simulink library "TQR_lib"  (Simulink 7.5)
settings: Solver=ode45  StartTime=0.0  StopTime=10.0  RelTol=1e-3
values from neighbouring files (symbols this model uses):
  p1_ACPI_PICFilDen1_na = Simulink.Parameter    [TQR_par.m]
  p1_ACPI_PICFilDen2_na = Simulink.Parameter    [TQR_par.m]
  p1_ACPI_PICFilDen3_na = Simulink.Parameter    [TQR_par.m]
  p1_ACPI_PICFilNum1_na = Simulink.Parameter    [TQR_par.m]
  p1_ACPI_PICFilNum2_na = Simulink.Parameter    [TQR_par.m]
  p1_ACPI_PICFilNum3_na = Simulink.Parameter    [TQR_par.m]
  pTQR_bar_BrkPOvrdRecoverThd_C = Simulink.Parameter    [TQR_par.m]
  pTQR_bar_BrkPOvrdVal_C = Simulink.Parameter    [TQR_par.m]
  pTQR_bar_ECrpTrqStrtPres_C = Simulink.Parameter    [TQR_par.m]
  pTQR_bar_MasterCylPres_CUR = Simulink.Parameter    [TQR_par.m]
  pTQR_bool_AccPedOvrdDsbl_C = Simulink.Parameter    [TQR_par.m]
  pTQR_bool_BrkPOvrdDsbl_C = Simulink.Parameter    [TQR_par.m]
  pTQR_bool_BrkRecupSrcSelSwt_C = Simulink.Parameter    [TQR_par.m]
  pTQR_bool_PICTqEna_C = Simulink.Parameter    [TQR_par.m]
  pTQR_bool_RecupEna_C = Simulink.Parameter    [TQR_par.m]
  pTQR_kmph_MaxVehSpd_C = Simulink.Parameter    [TQR_par.m]
  pTQR_kmph_MinVehSpd_C = Simulink.Parameter    [TQR_par.m]
  pTQR_kmph_VehSpd_TAB = Simulink.Parameter    [TQR_par.m]
  pTQR_kmph_VehSpdMaxDriving_TAB = Simulink.Parameter    [TQR_par.m]
  pTQR_kmph_VehSpdMaxReverse_TAB = Simulink.Parameter    [TQR_par.m]
  pTQR_kmph_VehSpdRednHi_CUR = Simulink.Parameter    [TQR_par.m]
  pTQR_kmph_VehSpdRednLo_CUR = Simulink.Parameter    [TQR_par.m]
  pTQR_Nm_ACCDelyOutTrq_C = Simulink.Parameter    [TQR_par.m]
  pTQR_Nm_ACCOutTrqLo_C = Simulink.Parameter    [TQR_par.m]
  pTQR_Nm_ACCOutTrqUp_C = Simulink.Parameter    [TQR_par.m]
  pTQR_Nm_BrkECrpTrq_TAB = Simulink.Parameter    [TQR_par.m]
  pTQR_Nm_MaxRecupTq_C = Simulink.Parameter    [TQR_par.m]
  pTQR_Nm_MotCtlrMaxTqLim_C = Simulink.Parameter    [TQR_par.m]
  pTQR_Nm_MotCtlrMinTqLim_C = Simulink.Parameter    [TQR_par.m]
  pTQR_Nm_PreloadTrq_C = Simulink.Parameter    [TQR_par.m]
  pTQR_Nm_PRNDLoTbl_MAP = Simulink.Parameter    [TQR_par.m]
  pTQR_Nm_RecupLoTbl_MAP = Simulink.Parameter    [TQR_par.m]
  pTQR_Nm_REDEVPRNDLoTbl_MAP = Simulink.Parameter    [TQR_par.m]
  pTQR_Nm_TqLimnUpprLim_C = Simulink.Parameter    [TQR_par.m]
  pTQR_Nmps_AccPedValLowrRateLim_CUR = Simulink.Parameter    [TQR_par.m]
  pTQR_Nmps_AccPedValUpprRateLim_CUR = Simulink.Parameter    [TQR_par.m]
  pTQR_Nmps_CrsCtlLowrRateLim_C = Simulink.Parameter    [TQR_par.m]
  pTQR_Nmps_CrsCtlUpprRateLim_C = Simulink.Parameter    [TQR_par.m]
  pTQR_Nmps_FltLowrRateLim_C = Simulink.Parameter    [TQR_par.m]
  pTQR_Nmps_FltUpprRateLim_C = Simulink.Parameter    [TQR_par.m]
  pTQR_Nmps_LowrRateLimLoTbl_TAB = Simulink.Parameter    [TQR_par.m]
  pTQR_Nmps_UpprRateLimLoTbl_TAB = Simulink.Parameter    [TQR_par.m]
  pTQR_pct_AccPedAcvThd_C = Simulink.Parameter    [TQR_par.m]
  pTQR_pct_AccPedOvrdRecThd_C = Simulink.Parameter    [TQR_par.m]
  pTQR_pct_AccPedOvrdVal_C = Simulink.Parameter    [TQR_par.m]
  pTQR_pct_AccPedThCC_C = Simulink.Parameter    [TQR_par.m]
  pTQR_pct_BrkPOvrdAccPedValThd_C = Simulink.Parameter    [TQR_par.m]
  pTQR_pct_PICAccPedValThd_C = Simulink.Parameter    [TQR_par.m]
  pTQR_r_BrkDwnFilterFac_C = Simulink.Parameter    [TQR_par.m]
  pTQR_r_BrkUpFilterFac_C = Simulink.Parameter    [TQR_par.m]
  pTQR_r_BrkWeightDsbl_C = Simulink.Parameter    [TQR_par.m]
  pTQR_r_BrkWeightFac_C = Simulink.Parameter    [TQR_par.m]
  pTQR_r_ECrpShfFilterFac_C = Simulink.Parameter    [TQR_par.m]
  pTQR_r_PICFilDen1_C = Simulink.Parameter    [TQR_par.m]
  pTQR_r_PICFilDen2_C = Simulink.Parameter    [TQR_par.m]
  pTQR_r_PICFilDen3_C = Simulink.Parameter    [TQR_par.m]
  pTQR_r_PICFilNum1_C = Simulink.Parameter    [TQR_par.m]
  pTQR_r_PICFilNum2_C = Simulink.Parameter    [TQR_par.m]
  pTQR_r_PICFilNum3_C = Simulink.Parameter    [TQR_par.m]
  pTQR_r_PreloadFilterFac_C = Simulink.Parameter    [TQR_par.m]
  pTQR_r_TrqDwnFilterFac_MAP = [ ... (first row only)    [TQR_par.m]
  pTQR_r_TrqUppFilterFac_MAP = [ ... (first row only)    [TQR_par.m]
  pTQR_r_VehSpdFilterFac_CUR = Simulink.Parameter    [TQR_par.m]
  pTQR_ratio_AccPedOvrdLoRate_C = Simulink.Parameter    [TQR_par.m]
  pTQR_ratio_AccPedOvrdUpRate_C = Simulink.Parameter    [TQR_par.m]
  pTQR_ratio_AccPedTqLimUpRate_C = Simulink.Parameter    [TQR_par.m]
  pTQR_ratio_BrkOvrAccPedGrdTh_C = Simulink.Parameter    [TQR_par.m]
  pTQR_ratio_BrkPOvrdLoRate_C = Simulink.Parameter    [TQR_par.m]
  pTQR_ratio_BrkPOvrdUpRate_C = Simulink.Parameter    [TQR_par.m]
  pTQR_ratio_PerfIdxGain_C = Simulink.Parameter    [TQR_par.m]
  pTQR_rpm_VehMoveSpdThrsh_C = Simulink.Parameter    [TQR_par.m]
  pTQR_rpm_VehStdStlSpdThrsh_C = Simulink.Parameter    [TQR_par.m]
  pTQR_s_AccPedActDly_C = Simulink.Parameter    [TQR_par.m]
  pTQR_s_ShfPreloadTrqTmrDly_C = Simulink.Parameter    [TQR_par.m]
  pTQR_s_ShfTrqTmrDly_C = Simulink.Parameter    [TQR_par.m]
  pTQR_s_SmplCyc_C = Simulink.Parameter    [TQR_par.m]
  pTQR_s_VehStdStlDly_C = Simulink.Parameter    [TQR_par.m]
undefined symbols (not defined in the file or in its folder): CrsCtlStsTyp, DiscIntNeverNeededParam, p_single_Minus_M, p_single_Zero_M, ShiftLvrPosnTyp
libraries: BaseOperationLib_Browser x214, simulink x11, PES_CZ_FAW x2, simulink_extras x2, A0EV_Lib1 x1
(part 1 of 2)
settings Model: Creator=wuaibin  LastModifiedBy=wuaibin

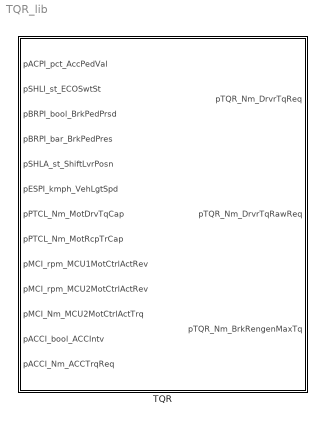
== system TQR_lib ==
  TQR : Subsystem  TreatAsAtomicUnit=on

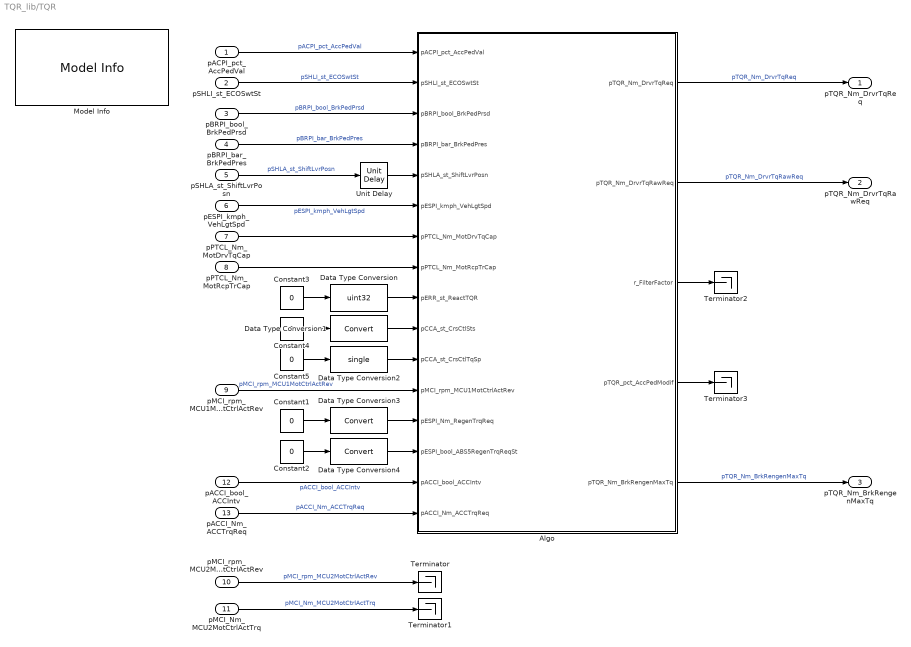
== system TQR_lib/TQR ==
  pACPI_pct_AccPedVal : Inport
  pSHLI_st_ECOSwtSt : Inport  Port=2
  pBRPI_bool_BrkPedPrsd : Inport  Port=3
  pBRPI_bar_BrkPedPres : Inport  Port=4
  pSHLA_st_ShiftLvrPosn : Inport  Port=5
  pESPI_kmph_VehLgtSpd : Inport  Port=6
  pPTCL_Nm_MotDrvTqCap : Inport  Port=7
  pPTCL_Nm_MotRcpTrCap : Inport  Port=8
  pMCI_rpm_MCU1MotCtrlActRev : Inport  Port=9
  pMCI_rpm_MCU2MotCtrlActRev : Inport  Port=10
  pMCI_Nm_MCU2MotCtrlActTrq : Inport  Port=11
  pACCI_bool_ACCIntv : Inport  Port=12
  pACCI_Nm_ACCTrqReq : Inport  Port=13
  Algo : Subsystem
  Constant{1..5} (5 alike) : Constant  Value=0  OutDataType=fixdt(1, 16)  OutScaling=2^0
  Data Type Conversion : DataTypeConversion  OutDataTypeMode=uint32  OutDataType=fixdt(1, 16)  OutScaling=2^0  OutDataTypeStr=uint32
  Data Type Conversion1 : DataTypeConversion  OutDataType=fixdt(1, 16)  OutScaling=2^0
  Data Type Conversion2 : DataTypeConversion  OutDataTypeMode=single  OutDataType=fixdt(1, 16)  OutScaling=2^0  OutDataTypeStr=single
  Data Type Conversion3 : DataTypeConversion  OutDataType=fixdt(1, 16)  OutScaling=2^0
  Data Type Conversion4 : DataTypeConversion  OutDataType=fixdt(1, 16)  OutScaling=2^0
  Model Info : simulink/Model-Wide Utilities/Model Info  SystemSampleTime=-1  InitialBlockCM=None  BlockCM=None  Frame=on  DisplayStringWithTags=Model Info\nCreated: %<Created>\nCreator: %<Creator>  HorizontalTextAlignment=Center  LeftAlignmentValue=0.5  SourceBlockDiagram=HQEV_HCU  TagMaxNumber=20
  Terminator{,1..3} (4 alike) : Terminator
  Unit Delay : BaseOperationLib_Browser/Discrete Unchanged /Unit Delay  X0=0  SampleTime=-1
  pTQR_Nm_DrvrTqReq : Outport  PortDimensions=1
  pTQR_Nm_DrvrTqRawReq : Outport  Port=2  PortDimensions=1
  pTQR_Nm_BrkRengenMaxTq : Outport  Port=3
  wires:
  pACCI_Nm_ACCTrqReq/1 -> Algo/16(pACCI_Nm_ACCTrqReq)  "pACCI_Nm_ACCTrqReq"
  pACCI_bool_ACCIntv/1 -> Algo/15(pACCI_bool_ACCIntv)  "pACCI_bool_ACCIntv"
  Unit Delay/1 -> Algo/5(pSHLA_st_ShiftLvrPosn)
  pMCI_rpm_MCU1MotCtrlActRev/1 -> Algo/12(pMCI_rpm_MCU1MotCtrlActRev)  "pMCI_rpm_MCU1MotCtrlActRev"
  pACPI_pct_AccPedVal/1 -> Algo/1(pACPI_pct_AccPedVal)  "pACPI_pct_AccPedVal"
  pSHLI_st_ECOSwtSt/1 -> Algo/2(pSHLI_st_ECOSwtSt)  "pSHLI_st_ECOSwtSt"
  pBRPI_bool_BrkPedPrsd/1 -> Algo/3(pBRPI_bool_BrkPedPrsd)  "pBRPI_bool_BrkPedPrsd"
  pBRPI_bar_BrkPedPres/1 -> Algo/4(pBRPI_bar_BrkPedPres)  "pBRPI_bar_BrkPedPres"
  pSHLA_st_ShiftLvrPosn/1 -> Unit Delay/1  "pSHLA_st_ShiftLvrPosn"
  pESPI_kmph_VehLgtSpd/1 -> Algo/6(pESPI_kmph_VehLgtSpd)  "pESPI_kmph_VehLgtSpd"
  Constant1/1 -> Data Type Conversion3/1
  Constant2/1 -> Data Type Conversion4/1
  Algo/1(pTQR_Nm_DrvrTqReq) -> pTQR_Nm_DrvrTqReq/1  "pTQR_Nm_DrvrTqReq"
  Algo/2(pTQR_Nm_DrvrTqRawReq) -> pTQR_Nm_DrvrTqRawReq/1  "pTQR_Nm_DrvrTqRawReq"
  Algo/5(pTQR_Nm_BrkRengenMaxTq) -> pTQR_Nm_BrkRengenMaxTq/1  "pTQR_Nm_BrkRengenMaxTq"
  pMCI_rpm_MCU2MotCtrlActRev/1 -> Terminator/1  "pMCI_rpm_MCU2MotCtrlActRev"
  pMCI_Nm_MCU2MotCtrlActTrq/1 -> Terminator1/1  "pMCI_Nm_MCU2MotCtrlActTrq"
  Algo/3(r_FilterFactor) -> Terminator2/1
  Algo/4(pTQR_pct_AccPedModif) -> Terminator3/1
  Constant3/1 -> Data Type Conversion/1
  Constant4/1 -> Data Type Conversion1/1
  Constant5/1 -> Data Type Conversion2/1
  Data Type Conversion/1 -> Algo/9(pERR_st_ReactTQR)
  Data Type Conversion1/1 -> Algo/10(pCCA_st_CrsCtlSts)
  Data Type Conversion2/1 -> Algo/11(pCCA_st_CrsCtlTqSp)
  Data Type Conversion3/1 -> Algo/13(pESPI_Nm_RegenTrqReq)
  Data Type Conversion4/1 -> Algo/14(pESPI_bool_ABS5RegenTrqReqSt)
  pPTCL_Nm_MotDrvTqCap/1 -> Algo/7(pPTCL_Nm_MotDrvTqCap)
  pPTCL_Nm_MotRcpTrCap/1 -> Algo/8(pPTCL_Nm_MotRcpTrCap)

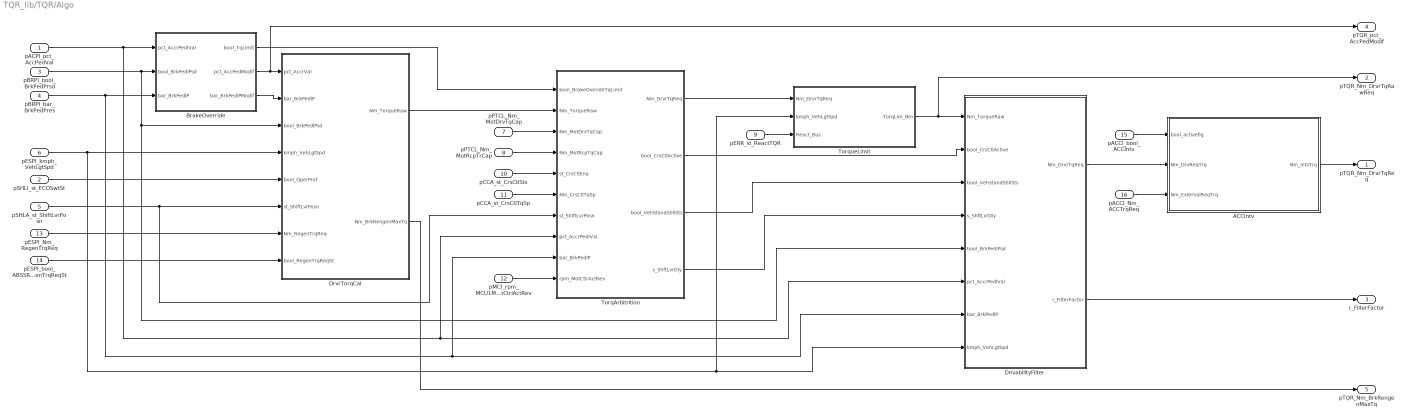
== system TQR_lib/TQR/Algo ==
  pACPI_pct_AccPedVal : Inport
  pSHLI_st_ECOSwtSt : Inport  Port=2
  pBRPI_bool_BrkPedPrsd : Inport  Port=3
  pBRPI_bar_BrkPedPres : Inport  Port=4
  pSHLA_st_ShiftLvrPosn : Inport  Port=5
  pESPI_kmph_VehLgtSpd : Inport  Port=6
  pPTCL_Nm_MotDrvTqCap : Inport  Port=7
  pPTCL_Nm_MotRcpTrCap : Inport  Port=8  PortDimensions=1
  pERR_st_ReactTQR : Inport  Port=9
  pCCA_st_CrsCtlSts : Inport  Port=10
  pCCA_st_CrsCtlTqSp : Inport  Port=11
  pMCI_rpm_MCU1MotCtrlActRev : Inport  Port=12
  pESPI_Nm_RegenTrqReq : Inport  Port=13  PortDimensions=1
  pESPI_bool_ABS5RegenTrqReqSt : Inport  Port=14  PortDimensions=1
  pACCI_bool_ACCIntv : Inport  Port=15
  pACCI_Nm_ACCTrqReq : Inport  Port=16
  ACCIntv : Subsystem
  BrakeOverride : Subsystem
  DrivabilityFilter : Subsystem
  DrvrTorqCal : Subsystem
  TorqArbitrition : Subsystem
  TorqueLimit : Subsystem
  pTQR_Nm_DrvrTqReq : Outport
  pTQR_Nm_DrvrTqRawReq : Outport  Port=2
  r_FilterFactor : Outport  Port=3
  pTQR_pct_AccPedModif : Outport  Port=4
  pTQR_Nm_BrkRengenMaxTq : Outport  Port=5
  wires:
  DrivabilityFilter/1(Nm_DrvrTqReq) -> ACCIntv/2(Nm_DrvReqTrq)
  ACCIntv/1(Nm_IntvTrq) -> pTQR_Nm_DrvrTqReq/1
  pACCI_Nm_ACCTrqReq/1 -> ACCIntv/3(Nm_ExternalReqTrq)
  pACCI_bool_ACCIntv/1 -> ACCIntv/1(bool_activeflg)
  pBRPI_bar_BrkPedPres/1 -> BrakeOverride/3(bar_BrkPedlP), DrivabilityFilter/7(bar_BrkPedlP), TorqArbitrition/9(bar_BrkPedlP)
  BrakeOverride/3(bar_BrkPedlPModif) -> DrvrTorqCal/2(bar_BrkPedlP)
  pERR_st_ReactTQR/1 -> TorqueLimit/3(React_Bus)
  pSHLI_st_ECOSwtSt/1 -> DrvrTorqCal/5(bool_OperProf)
  pESPI_kmph_VehLgtSpd/1 -> DrvrTorqCal/4(kmph_VehLgtSpd), DrivabilityFilter/8(kmph_VehLgtSpd), TorqueLimit/2(kmph_VehLgtSpd)
  pBRPI_bool_BrkPedPrsd/1 -> BrakeOverride/2(bool_BrkPedlPsd), DrvrTorqCal/3(bool_BrkPedlPsd), DrivabilityFilter/5(bool_BrkPedlPsd)
  pSHLA_st_ShiftLvrPosn/1 -> DrvrTorqCal/6(st_ShiftLvrPosn), TorqArbitrition/7(st_ShiftLvrPosn)
  TorqArbitrition/2(bool_CrsCtlActive) -> DrivabilityFilter/2(bool_CrsCtlActive)
  pCCA_st_CrsCtlTqSp/1 -> TorqArbitrition/6(Nm_CrsCtlTqSp)
  pCCA_st_CrsCtlSts/1 -> TorqArbitrition/5(st_CrsCtlEna)
  DrvrTorqCal/1(Nm_TorqueRaw) -> TorqArbitrition/2(Nm_TorqueRaw)
  BrakeOverride/2(pct_AccPedModif) -> DrvrTorqCal/1(pct_AccrVal), pTQR_pct_AccPedModif/1
  pACPI_pct_AccPedVal/1 -> BrakeOverride/1(pct_AccrPedlVal), DrivabilityFilter/6(pct_AccrPedlVal), TorqArbitrition/8(pct_AccrPedlVal)
  pPTCL_Nm_MotDrvTqCap/1 -> TorqArbitrition/3(Nm_MotDrvTqCap)
  pPTCL_Nm_MotRcpTrCap/1 -> TorqArbitrition/4(Nm_MotRcpTqCap)
  BrakeOverride/1(bool_TqLimit) -> TorqArbitrition/1(bool_BrakeOverideTqLimit)
  DrivabilityFilter/2(r_FilterFactor) -> r_FilterFactor/1
  pESPI_Nm_RegenTrqReq/1 -> DrvrTorqCal/7(Nm_RegenTrqReq)
  DrvrTorqCal/2(Nm_BrkRengenMaxTq) -> pTQR_Nm_BrkRengenMaxTq/1
  pESPI_bool_ABS5RegenTrqReqSt/1 -> DrvrTorqCal/8(bool_RegenTrqReqSt)
  pMCI_rpm_MCU1MotCtrlActRev/1 -> TorqArbitrition/10(rpm_MotCtlrActRev)
  TorqueLimit/1(TorqLim_Nm) -> DrivabilityFilter/1(Nm_TorqueRaw), pTQR_Nm_DrvrTqRawReq/1
  TorqArbitrition/1(Nm_DrvrTqReq) -> TorqueLimit/1(Nm_DrvrTqReq)
  TorqArbitrition/3(bool_VehStandStillSts) -> DrivabilityFilter/3(bool_VehStandStillSts)
  TorqArbitrition/4(s_ShftLvrDly) -> DrivabilityFilter/4(s_ShftLvrDly)

== system TQR_lib/TQR/Algo/ACCIntv ==
  bool_activeflg : Inport
  Nm_DrvReqTrq : Inport  Port=2
  Nm_ExternalReqTrq : Inport  Port=3
  Active : Subsystem
  Constant : BaseOperationLib_Browser/Sources&Sinks/Constant  Value=pTQR_Nm_ACCDelyOutTrq_C  OutMin=[]  OutMax=[]  OutDataType=fixdt(1, 16)  ConRadixGroup=Use specified scaling  OutScaling=2^0  OutDataTypeStr=Inherit: Inherit from 'Constant value'
  DeactiveDely : Subsystem
  Merge : Merge  Inputs=3
  Normal : Subsystem
  Unit Delay : BaseOperationLib_Browser/Discrete Unchanged /Unit Delay  X0=0  SampleTime=-1
  trq_arbitration : Stateflow chart  TreatAsAtomicUnit=on
  Nm_IntvTrq : Outport  OutDataType=fixdt(1, 16)  OutScaling=2^0
  wires:
  Constant/1 -> trq_arbitration/4(Nm_DelyOutTrq)
  Nm_ExternalReqTrq/1 -> Active/1(Nm_ExternalReqTrq)
  Unit Delay/1 -> DeactiveDely/2(Nm_FeedBackTrq), trq_arbitration/3(feedback_trq)
  Merge/1 -> Nm_IntvTrq/1, Unit Delay/1
  DeactiveDely/1(Nm_DeactiveDelyTrq) -> Merge/3
  Active/1(Nm_ActiveTrq) -> Merge/2
  Normal/1(Nm_Normal) -> Merge/1
  trq_arbitration/3(deactive_dely) -> DeactiveDely/Trigger
  trq_arbitration/2(active) -> Active/Trigger
  trq_arbitration/1(normal) -> Normal/Trigger
  Nm_DrvReqTrq/1 -> DeactiveDely/1(Nm_DrvReqTrq), Normal/1(Nm_DrvReqTrq), trq_arbitration/2(req_trq)
  bool_activeflg/1 -> trq_arbitration/1(active_flg)

== system TQR_lib/TQR/Algo/BrakeOverride ==
  pct_AccrPedlVal : Inport
  bool_BrkPedlPsd : Inport  Port=2
  bar_BrkPedlP : Inport  Port=3
  AccrPedlOverride : Subsystem
  Add1 : BaseOperationLib_Browser/Math Operations Changed/Sum  Inputs=-+  OutMin=[]  OutMax=[]  OutDataType=fixdt(1, 16)  OutScaling=2^0  OutDataTypeStr=Inherit: Inherit via back propagation
  BrkPOverride : Subsystem
  Chart : Stateflow chart  TreatAsAtomicUnit=on
  Constant8 : BaseOperationLib_Browser/Sources&Sinks/Constant  Value=pTQR_pct_BrkPOvrdAccPedValThd_C  OutMin=[]  OutMax=[]  OutDataType=fixdt(1, 16)  ConRadixGroup=Use specified scaling  OutScaling=2^0  OutDataTypeStr=Inherit: Inherit from 'Constant value'
  Convert4 : DataTypeConversion  OutDataType=fixdt(1, 16)  OutScaling=2^0
  Logical Operator2 : BaseOperationLib_Browser/Logic Operations Changed/Logical Operator  Operator=AND  Inputs=2  AllPortsSameDT=off  OutDataTypeMode=boolean  LogicDataType=PDT_Bool  OutDataTypeStr=boolean
  Relational Operator3 : BaseOperationLib_Browser/Logic Operations Changed/Relational Operator  Operator=>  LogicOutDataTypeMode=boolean  LogicDataType=PDT_Bool  OutDataTypeStr=boolean
  Second_order_derivative_filter : Subsystem
  Switch2 : BaseOperationLib_Browser/Signal Routing Changed/Switch  Criteria=u2 ~= 0  Threshold=0  OutMin=[]  OutMax=[]  OutDataType=fixdt(1,16,0)  OutScaling=[]
  Unit Delay : BaseOperationLib_Browser/Discrete Unchanged /Unit Delay  X0=0  SampleTime=-1
  bool_TqLimit : Outport
  pct_AccPedModif : Outport  Port=2
  bar_BrkPedlPModif : Outport  Port=3
  wires:
  Relational Operator3/1 -> Logical Operator2/2
  Constant8/1 -> Relational Operator3/2
  bar_BrkPedlP/1 -> Switch2/3, Add1/2
  Unit Delay/1 -> Switch2/1
  Switch2/1 -> Add1/1, Unit Delay/1
  Chart/2(bool_TqLimit) -> Logical Operator2/1, bool_TqLimit/1, AccrPedlOverride/3(bool_TqLimit)
  pct_AccrPedlVal/1 -> Relational Operator3/1, Chart/1(pct_AccrPedlVal), AccrPedlOverride/1(pct_AccrPedlIn), Second_order_derivative_filter/1(u_t)  "accr pedl"
  bool_BrkPedlPsd/1 -> Switch2/2, Chart/3(bool_BrkPedlPsd)  "brk pedl"
  Second_order_derivative_filter/1(Y_t) -> Convert4/1
  Chart/1(bool_OverrideActive) -> AccrPedlOverride/2(bool_OverrideSwitch)  "override active"
  AccrPedlOverride/1(AccrVal) -> pct_AccPedModif/1  "pTQR_pct_AccValMem"
  Logical Operator2/1 -> BrkPOverride/1(bool_OverrideSwitch)
  Add1/1 -> BrkPOverride/2(bar_PressureIn)
  BrkPOverride/1(bar_BrkPedlPModif) -> bar_BrkPedlPModif/1  "pDTR_bar_BrkPedPModifMem"
  Convert4/1 -> Chart/2(ratio_AccrPedlGrad)

== system TQR_lib/TQR/Algo/DrivabilityFilter ==
  Nm_TorqueRaw : Inport
  bool_CrsCtlActive : Inport  Port=2
  bool_VehStandStillSts : Inport  Port=3
  s_ShftLvrDly : Inport  Port=4
  bool_BrkPedlPsd : Inport  Port=5
  pct_AccrPedlVal : Inport  Port=6
  bar_BrkPedlP : Inport  Port=7
  kmph_VehLgtSpd : Inport  Port=8
  DrivingFilter : Subsystem
  TorqRateLimit : Subsystem
  Nm_DrvrTqReq : Outport
  r_FilterFactor : Outport  Port=2
  wires:
  pct_AccrPedlVal/1 -> TorqRateLimit/3(pct_AccrPedlVal), DrivingFilter/2(pct_AccrPedlVal)
  bool_CrsCtlActive/1 -> TorqRateLimit/2(bool_CrsCtlActive)
  TorqRateLimit/1(Nm_TorqRateLimit) -> DrivingFilter/1(Nm_TorqRateLimit)
  Nm_TorqueRaw/1 -> TorqRateLimit/1(Nm_TorqueRaw)
  bar_BrkPedlP/1 -> DrivingFilter/4(bar_BrkPedlP)
  bool_BrkPedlPsd/1 -> DrivingFilter/3(bool_BrkPedlPsd)
  kmph_VehLgtSpd/1 -> DrivingFilter/5(kmph_VehLgtSpd)
  s_ShftLvrDly/1 -> DrivingFilter/6(s_ShftLvrDly)
  bool_VehStandStillSts/1 -> DrivingFilter/7(bool_VehStandStillSts)
  DrivingFilter/2(r_DrivingFilterFactor) -> r_FilterFactor/1
  DrivingFilter/1(Nm_FilterTorqReq) -> Nm_DrvrTqReq/1

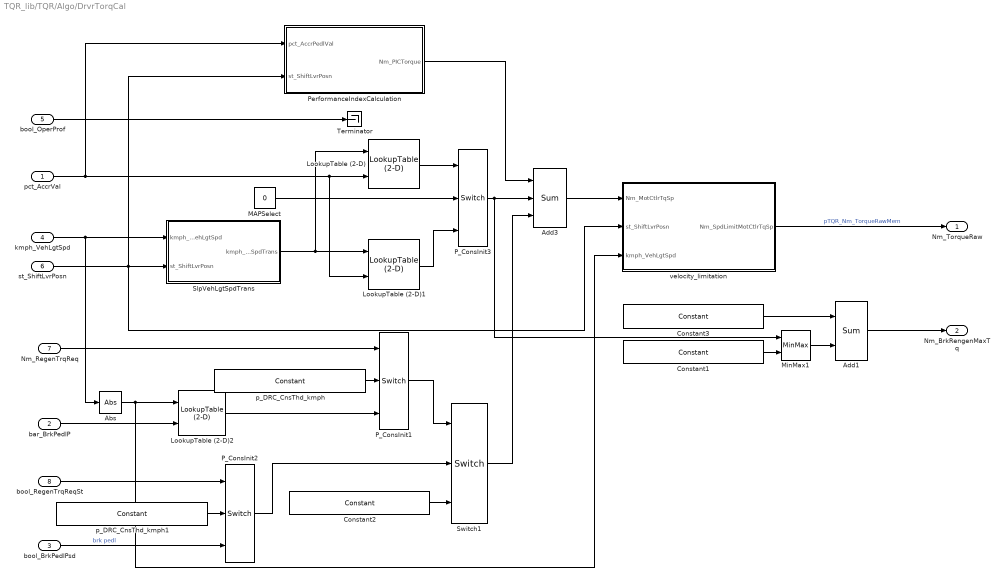
== system TQR_lib/TQR/Algo/DrvrTorqCal ==
  pct_AccrVal : Inport
  bar_BrkPedlP : Inport  Port=2
  bool_BrkPedlPsd : Inport  Port=3
  kmph_VehLgtSpd : Inport  Port=4
  bool_OperProf : Inport  Port=5
  st_ShiftLvrPosn : Inport  Port=6
  Nm_RegenTrqReq : Inport  Port=7  PortDimensions=1
  bool_RegenTrqReqSt : Inport  Port=8  PortDimensions=1
  Abs : BaseOperationLib_Browser/Math Operations Changed/Abs  OutMax=[]  OutDataType=fixdt(1, 16)  OutScaling=2^0
  Add1 : BaseOperationLib_Browser/Math Operations Changed/Sum  Inputs=+-  OutMin=[]  OutMax=[]  OutDataType=fixdt(1, 16)  OutScaling=2^0
  Add3 : BaseOperationLib_Browser/Math Operations Changed/Sum  Inputs=++-  OutMin=[]  OutMax=[]  OutDataType=fixdt(1, 16)  OutScaling=2^0
  Constant1 : BaseOperationLib_Browser/Sources&Sinks/Constant  Value=p_single_Zero_M  OutMin=[]  OutMax=[]  OutDataType=fixdt(1, 16)  ConRadixGroup=Use specified scaling  OutScaling=2^0  OutDataTypeStr=Inherit: Inherit from 'Constant value'
  Constant2 : BaseOperationLib_Browser/Sources&Sinks/Constant  Value=p_single_Zero_M  OutMin=[]  OutMax=[]  OutDataType=fixdt(1, 16)  ConRadixGroup=Use specified scaling  OutScaling=2^0  OutDataTypeStr=Inherit: Inherit from 'Constant value'
  Constant3 : BaseOperationLib_Browser/Sources&Sinks/Constant  Value=pTQR_Nm_MaxRecupTq_C  OutMin=[]  OutMax=[]  OutDataType=fixdt(1, 16)  ConRadixGroup=Use specified scaling  OutScaling=2^0  OutDataTypeStr=Inherit: Inherit from 'Constant value'
  LookupTable (2-D) : BaseOperationLib_Browser/Lookup Tables Changed/LookupTable (2-D)  RowIndex=pTQR_kmph_SpdLoTblVal_TABX  ColumnIndex=pTQR_pct_AccPedLoTblVal_TABY  Table=pTQR_Nm_PRNDLoTbl_MAP  LookUpMeth=Interpolation-Use End Values  OutMin=[]  OutMax=[]  OutDataType=fixdt(1, 16)  OutScaling=2^0  OutDataTypeStr=Inherit: Inherit via back propagation  SaturateOnIntegerOverflow=on
      settings: AttributesFormatString=X:%<RowIndex>\nY:%<ColumnIndex>\nTAB:%<Table>
  LookupTable (2-D)1 : BaseOperationLib_Browser/Lookup Tables Changed/LookupTable (2-D)  RowIndex=pTQR_kmph_RedEVSpdLoTblVal_TABX  ColumnIndex=pTQR_pct_AccPedLoTblVal_TABY  Table=pTQR_Nm_REDEVPRNDLoTbl_MAP  LookUpMeth=Interpolation-Use End Values  OutMin=[]  OutMax=[]  OutDataType=fixdt(1, 16)  OutScaling=2^0  OutDataTypeStr=Inherit: Inherit via back propagation  SaturateOnIntegerOverflow=on
      settings: AttributesFormatString=X:%<RowIndex>\nY:%<ColumnIndex>\nTAB:%<Table>
  LookupTable (2-D)2 : BaseOperationLib_Browser/Lookup Tables Changed/LookupTable (2-D)  RowIndex=pTQR_kmph_RecupSpdLoTblVal_TABX  ColumnIndex=pTQR_bar_BrkPedlLoTblVal_TABY  Table=pTQR_Nm_RecupLoTbl_MAP  LookUpMeth=Interpolation-Use End Values  OutMin=[]  OutMax=[]  OutDataType=fixdt(1, 16)  OutScaling=2^0  OutDataTypeStr=Inherit: Inherit via back propagation  SaturateOnIntegerOverflow=on
      settings: AttributesFormatString=X:%<RowIndex>\nY:%<ColumnIndex>\nTAB:%<Table>
  MAPSelect : Constant  Value=0  OutDataType=fixdt(1, 16)  OutScaling=2^0
  MinMax1 : BaseOperationLib_Browser/Math Operations Changed/MinMax  Function=min  Inputs=2  InputSameDT=on  OutMin=[]  OutMax=[]  OutDataType=fixdt(1, 16)  OutScaling=2^0  SaturateOnIntegerOverflow=on
  P_ConsInit1 : BaseOperationLib_Browser/Signal Routing Changed/Switch  Criteria=u2 > Threshold  Threshold=0  OutMin=[]  OutMax=[]  OutDataType=fixdt(1,16,0)  OutScaling=[]  OutDataTypeStr=Inherit: Inherit via back propagation
  P_ConsInit2 : BaseOperationLib_Browser/Signal Routing Changed/Switch  Criteria=u2 > Threshold  Threshold=0  OutMin=[]  OutMax=[]  OutDataType=fixdt(1,16,0)  OutScaling=[]  OutDataTypeStr=Inherit: Inherit via back propagation
  P_ConsInit3 : BaseOperationLib_Browser/Signal Routing Changed/Switch  Criteria=u2 > Threshold  Threshold=0  OutMin=[]  OutMax=[]  OutDataType=fixdt(1,16,0)  OutScaling=[]  OutDataTypeStr=Inherit: Inherit via back propagation
  PerformanceIndexCalculation : Subsystem
  SlpVehLgtSpdTrans : Subsystem
  Switch1 : BaseOperationLib_Browser/Signal Routing Changed/Switch  Criteria=u2 ~= 0  Threshold=0  OutMin=[]  OutMax=[]  OutDataType=fixdt(1,16,0)  OutScaling=[]
  Terminator : Terminator
  p_DRC_CnsThd_kmph : BaseOperationLib_Browser/Sources&Sinks/Constant  Value=pTQR_bool_BrkRecupSrcSelSwt_C  OutMin=[]  OutMax=[]  OutDataTypeMode=boolean  OutDataType=fixdt(1, 16)  ConRadixGroup=Use specified scaling  OutScaling=2^0  OutDataTypeStr=boolean
  p_DRC_CnsThd_kmph1 : BaseOperationLib_Browser/Sources&Sinks/Constant  Value=pTQR_bool_BrkRecupSrcSelSwt_C  OutMin=[]  OutMax=[]  OutDataTypeMode=boolean  OutDataType=fixdt(1, 16)  ConRadixGroup=Use specified scaling  OutScaling=2^0  OutDataTypeStr=boolean
  velocity_limitation : Subsystem
  Nm_TorqueRaw : Outport
  Nm_BrkRengenMaxTq : Outport  Port=2
  wires:
  MAPSelect/1 -> P_ConsInit3/2
  LookupTable (2-D)1/1 -> P_ConsInit3/3
  LookupTable (2-D)/1 -> P_ConsInit3/1
  P_ConsInit3/1 -> MinMax1/1, Add3/2
  Constant2/1 -> Switch1/3
  bar_BrkPedlP/1 -> LookupTable (2-D)2/2
  pct_AccrVal/1 -> LookupTable (2-D)1/2, LookupTable (2-D)/2, PerformanceIndexCalculation/1(pct_AccrPedlVal)
  kmph_VehLgtSpd/1 -> Abs/1, SlpVehLgtSpdTrans/1(kmph_VehLgtSpd)
  SlpVehLgtSpdTrans/1(kmph_SlpVehLgtSpdTrans) -> LookupTable (2-D)1/1, LookupTable (2-D)/1
  Abs/1 -> LookupTable (2-D)2/1, velocity_limitation/3(kmph_VehLgtSpd)
  Add3/1 -> velocity_limitation/1(Nm_MotCtlrTqSp)
  PerformanceIndexCalculation/1(Nm_PICTorque) -> Add3/1
  Switch1/1 -> Add3/3
  velocity_limitation/1(Nm_SpdLimitMotCtlrTqSp) -> Nm_TorqueRaw/1  "pTQR_Nm_TorqueRawMem"
  p_DRC_CnsThd_kmph/1 -> P_ConsInit1/2
  LookupTable (2-D)2/1 -> P_ConsInit1/3
  P_ConsInit1/1 -> Switch1/1
  Constant3/1 -> Add1/1
  Nm_RegenTrqReq/1 -> P_ConsInit1/1
  Constant1/1 -> MinMax1/2
  MinMax1/1 -> Add1/2
  Add1/1 -> Nm_BrkRengenMaxTq/1
  p_DRC_CnsThd_kmph1/1 -> P_ConsInit2/2
  P_ConsInit2/1 -> Switch1/2
  bool_RegenTrqReqSt/1 -> P_ConsInit2/1
  bool_BrkPedlPsd/1 -> P_ConsInit2/3  "brk pedl"
  bool_OperProf/1 -> Terminator/1
  st_ShiftLvrPosn/1 -> SlpVehLgtSpdTrans/2(st_ShiftLvrPosn), PerformanceIndexCalculation/2(st_ShiftLvrPosn), velocity_limitation/2(st_ShiftLvrPosn)

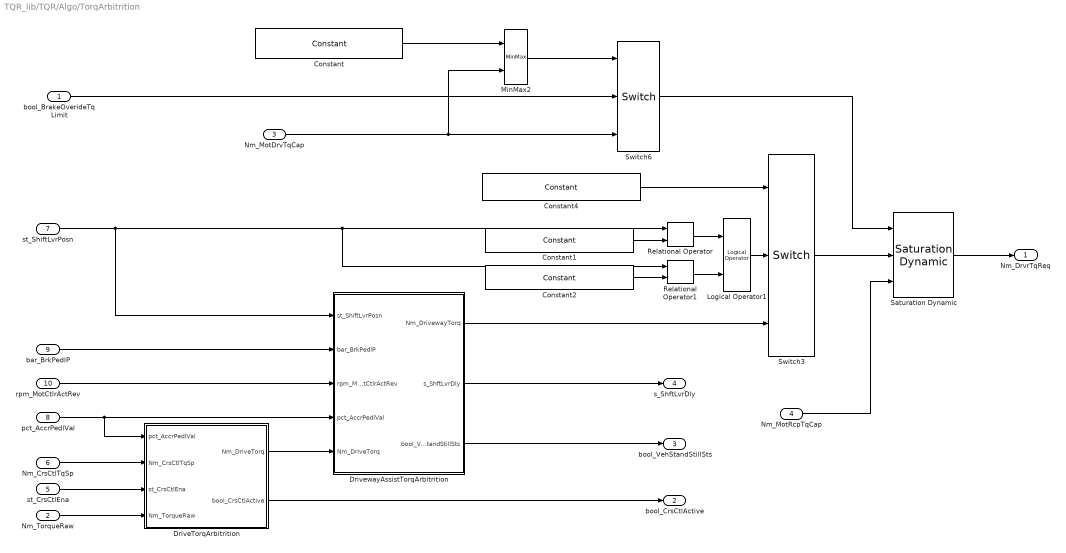
== system TQR_lib/TQR/Algo/TorqArbitrition ==
  bool_BrakeOverideTqLimit : Inport
  Nm_TorqueRaw : Inport  Port=2
  Nm_MotDrvTqCap : Inport  Port=3
  Nm_MotRcpTqCap : Inport  Port=4
  st_CrsCtlEna : Inport  Port=5
  Nm_CrsCtlTqSp : Inport  Port=6
  st_ShiftLvrPosn : Inport  Port=7
  pct_AccrPedlVal : Inport  Port=8
  bar_BrkPedlP : Inport  Port=9
  rpm_MotCtlrActRev : Inport  Port=10
  Constant : BaseOperationLib_Browser/Sources&Sinks/Constant  Value=pTQR_Nm_TqLimnUpprLim_C  OutMin=[]  OutMax=[]  OutDataType=fixdt(1, 16)  ConRadixGroup=Use specified scaling  OutScaling=2^0  OutDataTypeStr=Inherit: Inherit from 'Constant value'
  Constant1 : BaseOperationLib_Browser/Sources&Sinks/Constant  Value=uint8(ShiftLvrPosnTyp.SHL_N)  OutMin=[]  OutMax=[]  OutDataType=fixdt(1, 16)  ConRadixGroup=Use specified scaling  OutScaling=2^0  OutDataTypeStr=Inherit: Inherit from 'Constant value'
  Constant2 : BaseOperationLib_Browser/Sources&Sinks/Constant  Value=uint8(ShiftLvrPosnTyp.SHL_P)  OutMin=[]  OutMax=[]  OutDataType=fixdt(1, 16)  ConRadixGroup=Use specified scaling  OutScaling=2^0  OutDataTypeStr=Inherit: Inherit from 'Constant value'
  Constant4 : BaseOperationLib_Browser/Sources&Sinks/Constant  Value=p_single_Zero_M  OutMin=[]  OutMax=[]  OutDataType=fixdt(1, 16)  ConRadixGroup=Use specified scaling  OutScaling=2^0  OutDataTypeStr=Inherit: Inherit from 'Constant value'
  DriveTorqArbitrition : Subsystem
  DrivewayAssistTorqArbitrition : Subsystem
  Logical Operator1 : BaseOperationLib_Browser/Logic Operations Changed/Logical Operator  Operator=OR  Inputs=2  AllPortsSameDT=off  OutDataTypeMode=boolean  LogicDataType=PDT_Bool  OutDataTypeStr=boolean
  MinMax2 : BaseOperationLib_Browser/Math Operations Changed/MinMax  Function=min  Inputs=2  OutMin=[]  OutMax=[]  OutDataType=fixdt(1, 16)  OutScaling=2^0
  Relational Operator : BaseOperationLib_Browser/Logic Operations Changed/Relational Operator  Operator===  InputSameDT=on  LogicOutDataTypeMode=Specify via dialog  LogicDataType=PDT_Bool  OutDataTypeStr=PDT_Bool
  Relational Operator1 : BaseOperationLib_Browser/Logic Operations Changed/Relational Operator  Operator===  InputSameDT=on  LogicOutDataTypeMode=Specify via dialog  LogicDataType=PDT_Bool  OutDataTypeStr=PDT_Bool
  Saturation Dynamic : BaseOperationLib_Browser/Discontinuities Unchanged/Saturation Dynamic  SystemSampleTime=-1  OutMin=[]  OutMax=[]  OutDataTypeStr=Inherit: Same as second input  OutDataType=fixdt(1, 16)  OutScaling=2^-10  DoSatur=off
  Switch3 : BaseOperationLib_Browser/Signal Routing Changed/Switch  Criteria=u2 ~= 0  Threshold=0  OutMin=[]  OutMax=[]  OutDataType=fixdt(1,16,0)  OutScaling=[]
  Switch6 : BaseOperationLib_Browser/Signal Routing Changed/Switch  Criteria=u2 ~= 0  Threshold=0  OutMin=[]  OutMax=[]  OutDataType=fixdt(1,16,0)  OutScaling=[]
  Nm_DrvrTqReq : Outport
  bool_CrsCtlActive : Outport  Port=2
  bool_VehStandStillSts : Outport  Port=3
  s_ShftLvrDly : Outport  Port=4  PortDimensions=1  OutDataType=fixdt(1, 16)  OutScaling=2^0
  wires:
  Logical Operator1/1 -> Switch3/2
  DriveTorqArbitrition/1(Nm_DriveTorq) -> DrivewayAssistTorqArbitrition/5(Nm_DriveTorq)
  DrivewayAssistTorqArbitrition/1(Nm_DrivewayTorq) -> Switch3/3
  Constant4/1 -> Switch3/1
  pct_AccrPedlVal/1 -> DrivewayAssistTorqArbitrition/4(pct_AccrPedlVal), DriveTorqArbitrition/1(pct_AccrPedlVal)
  st_CrsCtlEna/1 -> DriveTorqArbitrition/3(st_CrsCtlEna)
  Saturation Dynamic/1 -> Nm_DrvrTqReq/1
  st_ShiftLvrPosn/1 -> Relational Operator/1, Relational Operator1/1, DrivewayAssistTorqArbitrition/1(st_ShiftLvrPosn)
  Constant1/1 -> Relational Operator/2
  Relational Operator/1 -> Logical Operator1/1
  Relational Operator1/1 -> Logical Operator1/2
  Constant2/1 -> Relational Operator1/2
  Switch3/1 -> Saturation Dynamic/2
  Nm_MotRcpTqCap/1 -> Saturation Dynamic/3
  Switch6/1 -> Saturation Dynamic/1
  MinMax2/1 -> Switch6/1
  Constant/1 -> MinMax2/1
  bool_BrakeOverideTqLimit/1 -> Switch6/2
  DriveTorqArbitrition/2(bool_CrsCtlActive) -> bool_CrsCtlActive/1
  Nm_MotDrvTqCap/1 -> Switch6/3, MinMax2/2
  DrivewayAssistTorqArbitrition/2(s_ShftLvrDly) -> s_ShftLvrDly/1
  bar_BrkPedlP/1 -> DrivewayAssistTorqArbitrition/2(bar_BrkPedlP)
  rpm_MotCtlrActRev/1 -> DrivewayAssistTorqArbitrition/3(rpm_MotCtlrActRev)
  DrivewayAssistTorqArbitrition/3(bool_VehStandStillSts) -> bool_VehStandStillSts/1
  Nm_CrsCtlTqSp/1 -> DriveTorqArbitrition/2(Nm_CrsCtlTqSp)
  Nm_TorqueRaw/1 -> DriveTorqArbitrition/4(Nm_TorqueRaw)

== system TQR_lib/TQR/Algo/TorqueLimit ==
  Nm_DrvrTqReq : Inport
  kmph_VehLgtSpd : Inport  Port=2
  React_Bus : Inport  Port=3
  Constant5 : BaseOperationLib_Browser/Sources&Sinks/Constant  Value=pTQR_Nmps_FltUpprRateLim_C  OutMin=[]  OutMax=[]  OutDataType=fixdt(1, 16)  ConRadixGroup=Use specified scaling  OutScaling=2^0  OutDataTypeStr=Inherit: Inherit from 'Constant value'
  Constant6 : BaseOperationLib_Browser/Sources&Sinks/Constant  Value=pTQR_Nmps_FltLowrRateLim_C  OutMin=[]  OutMax=[]  OutDataType=fixdt(1, 16)  ConRadixGroup=Use specified scaling  OutScaling=2^0  OutDataTypeStr=Inherit: Inherit from 'Constant value'
  Rate Limiter Dynamic1 : BaseOperationLib_Browser/Discontinuities Unchanged/Rate Limiter Dynamic  SystemSampleTime=-1
  no_recuperation : Subsystem
  torque_reduction : Subsystem
  velocity_reduction : Subsystem
  TorqLim_Nm : Outport
  wires:
  Rate Limiter Dynamic1/1 -> TorqLim_Nm/1
  no_recuperation/1(Nm_NoRecupTorq) -> Rate Limiter Dynamic1/2
  Constant5/1 -> Rate Limiter Dynamic1/1
  Constant6/1 -> Rate Limiter Dynamic1/3
  Nm_DrvrTqReq/1 -> velocity_reduction/1(Nm_MotCtlrTqSp)
  kmph_VehLgtSpd/1 -> velocity_reduction/2(kmph_VehLgtSpd)
  React_Bus/1 -> velocity_reduction/3(React_Bus), torque_reduction/2(React_Bus), no_recuperation/2(React_Bus)
  torque_reduction/1(Nm_ReductionTorq) -> no_recuperation/1(Nm_ReductionTorq)
  velocity_reduction/1(Nm_VelReducTrq) -> torque_reduction/1(Nm_VelReducTorq)

== system TQR_lib/TQR/Algo/ACCIntv/Active ==
  Nm_ExternalReqTrq : Inport  OutDataType=fixdt(1, 16)  OutScaling=2^0
  function : TriggerPort  TriggerType=function-call
  Nm_ActiveTrq : Outport  OutDataType=fixdt(1, 16)  OutScaling=2^0
  wires:
  Nm_ExternalReqTrq/1 -> Nm_ActiveTrq/1

== system TQR_lib/TQR/Algo/ACCIntv/DeactiveDely ==
  Nm_DrvReqTrq : Inport  OutDataType=fixdt(1, 16)  OutScaling=2^0
  Nm_FeedBackTrq : Inport  Port=2  OutDataType=fixdt(1, 16)  OutScaling=2^0
  function : TriggerPort  TriggerType=function-call
  Constant : BaseOperationLib_Browser/Sources&Sinks/Constant  Value=pTQR_Nm_ACCOutTrqUp_C  OutMin=[]  OutMax=[]  OutDataType=fixdt(1, 16)  ConRadixGroup=Use specified scaling  OutScaling=2^0  OutDataTypeStr=Inherit: Inherit from 'Constant value'
  Constant1 : BaseOperationLib_Browser/Sources&Sinks/Constant  Value=pTQR_Nm_ACCOutTrqLo_C  OutMin=[]  OutMax=[]  OutDataType=fixdt(1, 16)  ConRadixGroup=Use specified scaling  OutScaling=2^0  OutDataTypeStr=Inherit: Inherit from 'Constant value'
  RampLim : A0EV_Lib1/Filter & Ramp/RampLim  SystemSampleTime=-1
  Nm_DeactiveDelyTrq : Outport  OutDataType=fixdt(1, 16)  OutScaling=2^0
  wires:
  Constant1/1 -> RampLim/4
  Constant/1 -> RampLim/3
  RampLim/1 -> Nm_DeactiveDelyTrq/1
  Nm_FeedBackTrq/1 -> RampLim/2
  Nm_DrvReqTrq/1 -> RampLim/1

== system TQR_lib/TQR/Algo/ACCIntv/Normal ==
  Nm_DrvReqTrq : Inport  OutDataType=fixdt(1, 16)  OutScaling=2^0
  function : TriggerPort  TriggerType=function-call
  Nm_Normal : Outport  OutDataType=fixdt(1, 16)  OutScaling=2^0
  wires:
  Nm_DrvReqTrq/1 -> Nm_Normal/1

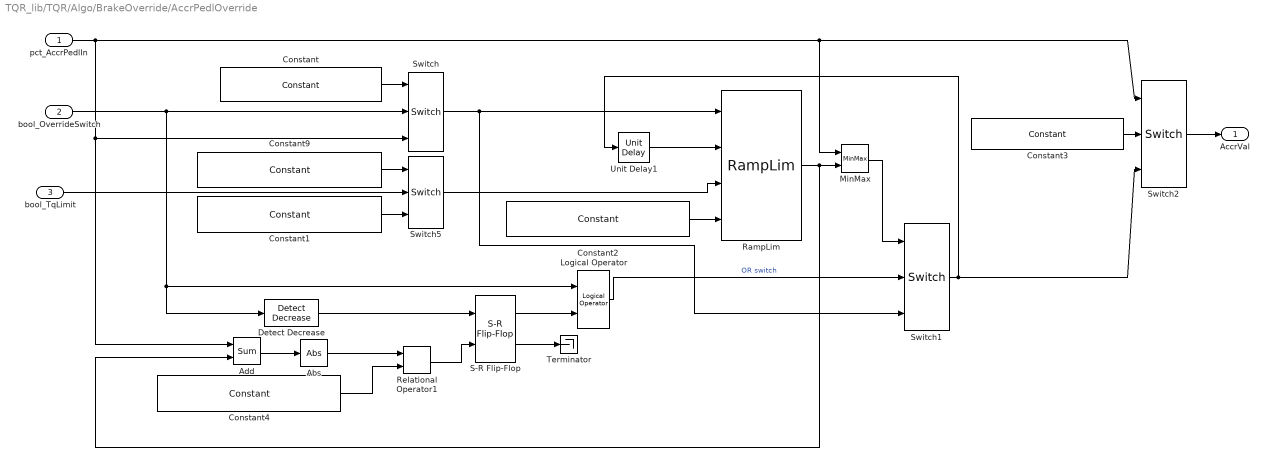
== system TQR_lib/TQR/Algo/BrakeOverride/AccrPedlOverride ==
  pct_AccrPedlIn : Inport
  bool_OverrideSwitch : Inport  Port=2
  bool_TqLimit : Inport  Port=3
  Abs : BaseOperationLib_Browser/Math Operations Changed/Abs  OutMax=[]  OutDataType=fixdt(1, 16)  OutScaling=2^0
  Add : BaseOperationLib_Browser/Math Operations Changed/Sum  Inputs=+-  OutMin=[]  OutMax=[]  OutDataType=fixdt(1, 16)  OutScaling=2^0
  Constant : BaseOperationLib_Browser/Sources&Sinks/Constant  Value=pTQR_pct_AccPedOvrdVal_C  OutMin=[]  OutMax=[]  OutDataType=fixdt(1, 16)  ConRadixGroup=Use specified scaling  OutScaling=2^0  OutDataTypeStr=Inherit: Inherit from 'Constant value'
  Constant1 : BaseOperationLib_Browser/Sources&Sinks/Constant  Value=pTQR_ratio_AccPedOvrdUpRate_C  OutMin=[]  OutMax=[]  OutDataType=fixdt(1, 16)  ConRadixGroup=Use specified scaling  OutScaling=2^0  OutDataTypeStr=Inherit: Inherit from 'Constant value'
  Constant2 : BaseOperationLib_Browser/Sources&Sinks/Constant  Value=pTQR_ratio_AccPedOvrdLoRate_C  OutMin=[]  OutMax=[]  OutDataType=fixdt(1, 16)  ConRadixGroup=Use specified scaling  OutScaling=2^0  OutDataTypeStr=Inherit: Inherit from 'Constant value'
  Constant3 : BaseOperationLib_Browser/Sources&Sinks/Constant  Value=pTQR_bool_AccPedOvrdDsbl_C  OutMin=[]  OutMax=[]  OutDataType=fixdt(1, 16)  ConRadixGroup=Use specified scaling  OutScaling=2^0  OutDataTypeStr=Inherit: Inherit from 'Constant value'
  Constant4 : BaseOperationLib_Browser/Sources&Sinks/Constant  Value=pTQR_pct_AccPedOvrdRecThd_C  OutMin=[]  OutMax=[]  OutDataType=fixdt(1, 16)  ConRadixGroup=Use specified scaling  OutScaling=2^0  OutDataTypeStr=Inherit: Inherit from 'Constant value'
  Constant9 : BaseOperationLib_Browser/Sources&Sinks/Constant  Value=pTQR_ratio_AccPedTqLimUpRate_C  OutMin=[]  OutMax=[]  OutDataType=fixdt(1, 16)  ConRadixGroup=Use specified scaling  OutScaling=2^0  OutDataTypeStr=Inherit: Inherit from 'Constant value'
  Detect Decrease : PES_CZ_FAW/Math_and_Discrete/Detect Decrease  SystemSampleTime=-1  vinit=0.0
  Logical Operator : BaseOperationLib_Browser/Logic Operations Changed/Logical Operator  Operator=OR  Inputs=2  AllPortsSameDT=off  OutDataTypeMode=boolean  LogicDataType=PDT_Bool  OutDataTypeStr=boolean
  MinMax : BaseOperationLib_Browser/Math Operations Changed/MinMax  Function=min  Inputs=2  OutMin=[]  OutMax=[]  OutDataType=fixdt(1, 16)  OutScaling=2^0
  RampLim : BaseOperationLib_Browser/Discontinuities Unchanged/RampLim  SystemSampleTime=-1
  Relational Operator1 : BaseOperationLib_Browser/Logic Operations Changed/Relational Operator  Operator=<  LogicOutDataTypeMode=boolean  LogicDataType=PDT_Bool  OutDataTypeStr=boolean
  S-R Flip-Flop : simulink_extras/Flip Flops/S-R Flip-Flop  SystemSampleTime=-1  initial_condition=0
  Switch{,1..2,5} (4 alike) : BaseOperationLib_Browser/Signal Routing Changed/Switch  Criteria=u2 ~= 0  Threshold=0  OutMin=[]  OutMax=[]  OutDataType=fixdt(1,16,0)  OutScaling=[]
  Terminator : Terminator
  Unit Delay1 : BaseOperationLib_Browser/Discrete Unchanged /Unit Delay  X0=0  SampleTime=-1
  AccrVal : Outport
  wires:
  Logical Operator/1 -> Switch1/2  "OR switch"
  Constant4/1 -> Relational Operator1/2
  Abs/1 -> Relational Operator1/1
  Add/1 -> Abs/1
  RampLim/1 -> Add/2, MinMax/2
  Switch/1 -> Switch1/3, RampLim/1
  Constant/1 -> Switch/1
  bool_OverrideSwitch/1 -> Switch/2, Logical Operator/1, Detect Decrease/1
  Switch1/1 -> Unit Delay1/1, Switch2/3
  Relational Operator1/1 -> S-R Flip-Flop/2
  S-R Flip-Flop/1 -> Logical Operator/2
  S-R Flip-Flop/2 -> Terminator/1
  Detect Decrease/1 -> S-R Flip-Flop/1
  MinMax/1 -> Switch1/1
  Unit Delay1/1 -> RampLim/2
  Constant2/1 -> RampLim/4
  Switch5/1 -> RampLim/3
  Constant1/1 -> Switch5/3
  Constant9/1 -> Switch5/1
  pct_AccrPedlIn/1 -> Add/1, Switch/3, MinMax/1, Switch2/1
  bool_TqLimit/1 -> Switch5/2
  Switch2/1 -> AccrVal/1
  Constant3/1 -> Switch2/2

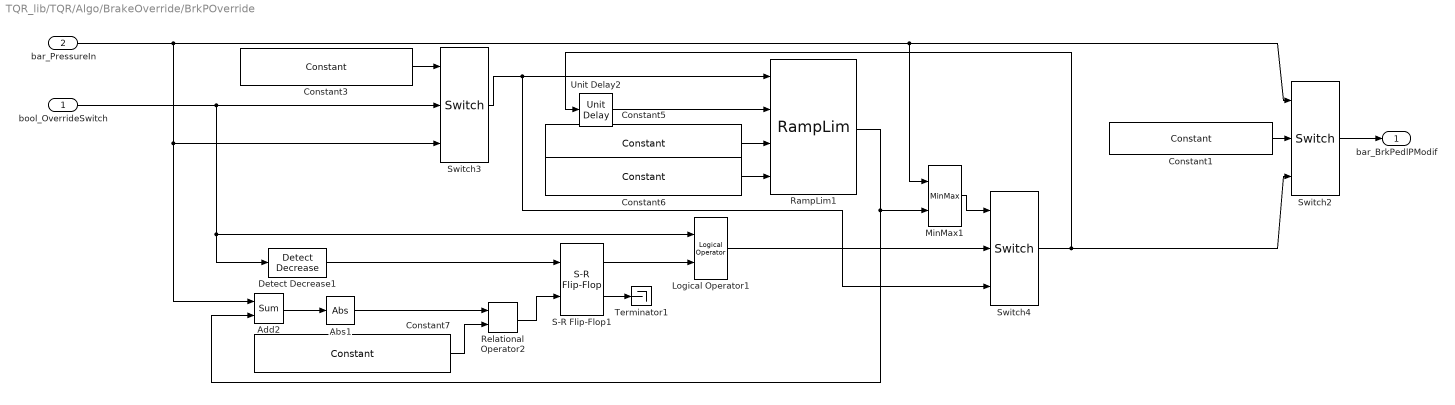
== system TQR_lib/TQR/Algo/BrakeOverride/BrkPOverride ==
  bool_OverrideSwitch : Inport
  bar_PressureIn : Inport  Port=2
  Abs1 : BaseOperationLib_Browser/Math Operations Changed/Abs  OutMax=[]  OutDataType=fixdt(1, 16)  OutScaling=2^0
  Add2 : BaseOperationLib_Browser/Math Operations Changed/Sum  Inputs=+-  OutMin=[]  OutMax=[]  OutDataType=fixdt(1, 16)  OutScaling=2^0
  Constant1 : BaseOperationLib_Browser/Sources&Sinks/Constant  Value=pTQR_bool_BrkPOvrdDsbl_C  OutMin=[]  OutMax=[]  OutDataType=fixdt(1, 16)  ConRadixGroup=Use specified scaling  OutScaling=2^0  OutDataTypeStr=Inherit: Inherit from 'Constant value'
  Constant3 : BaseOperationLib_Browser/Sources&Sinks/Constant  Value=pTQR_bar_BrkPOvrdVal_C  OutMin=[]  OutMax=[]  OutDataType=fixdt(1, 16)  ConRadixGroup=Use specified scaling  OutScaling=2^0  OutDataTypeStr=Inherit: Inherit from 'Constant value'
  Constant5 : BaseOperationLib_Browser/Sources&Sinks/Constant  Value=pTQR_ratio_BrkPOvrdUpRate_C  OutMin=[]  OutMax=[]  OutDataType=fixdt(1, 16)  ConRadixGroup=Use specified scaling  OutScaling=2^0  OutDataTypeStr=Inherit: Inherit from 'Constant value'
  Constant6 : BaseOperationLib_Browser/Sources&Sinks/Constant  Value=pTQR_ratio_BrkPOvrdLoRate_C  OutMin=[]  OutMax=[]  OutDataType=fixdt(1, 16)  ConRadixGroup=Use specified scaling  OutScaling=2^0  OutDataTypeStr=Inherit: Inherit from 'Constant value'
  Constant7 : BaseOperationLib_Browser/Sources&Sinks/Constant  Value=pTQR_bar_BrkPOvrdRecoverThd_C  OutMin=[]  OutMax=[]  OutDataType=fixdt(1, 16)  ConRadixGroup=Use specified scaling  OutScaling=2^0  OutDataTypeStr=Inherit: Inherit from 'Constant value'
  Detect Decrease1 : PES_CZ_FAW/Math_and_Discrete/Detect Decrease  SystemSampleTime=-1  vinit=0.0
  Logical Operator1 : BaseOperationLib_Browser/Logic Operations Changed/Logical Operator  Operator=OR  Inputs=2  AllPortsSameDT=off  OutDataTypeMode=boolean  LogicDataType=PDT_Bool  OutDataTypeStr=boolean
  MinMax1 : BaseOperationLib_Browser/Math Operations Changed/MinMax  Function=min  Inputs=2  OutMin=[]  OutMax=[]  OutDataType=fixdt(1, 16)  OutScaling=2^0
  RampLim1 : BaseOperationLib_Browser/Discontinuities Unchanged/RampLim  SystemSampleTime=-1
  Relational Operator2 : BaseOperationLib_Browser/Logic Operations Changed/Relational Operator  Operator=<  LogicOutDataTypeMode=boolean  LogicDataType=PDT_Bool  OutDataTypeStr=boolean
  S-R Flip-Flop1 : simulink_extras/Flip Flops/S-R Flip-Flop  SystemSampleTime=-1  initial_condition=0
  Switch2 : BaseOperationLib_Browser/Signal Routing Changed/Switch  Criteria=u2 ~= 0  Threshold=0  OutMin=[]  OutMax=[]  OutDataType=fixdt(1,16,0)  OutScaling=[]
  Switch3 : BaseOperationLib_Browser/Signal Routing Changed/Switch  Criteria=u2 ~= 0  Threshold=0  OutMin=[]  OutMax=[]  OutDataType=fixdt(1,16,0)  OutScaling=[]
  Switch4 : BaseOperationLib_Browser/Signal Routing Changed/Switch  Criteria=u2 ~= 0  Threshold=0  OutMin=[]  OutMax=[]  OutDataType=fixdt(1,16,0)  OutScaling=[]
  Terminator1 : Terminator
  Unit Delay2 : BaseOperationLib_Browser/Discrete Unchanged /Unit Delay  X0=0  SampleTime=-1
  bar_BrkPedlPModif : Outport
  wires:
  Switch4/1 -> Unit Delay2/1, Switch2/3
  bar_PressureIn/1 -> Switch3/3, Add2/1, Switch2/1, MinMax1/1
  Logical Operator1/1 -> Switch4/2
  Constant7/1 -> Relational Operator2/2
  Abs1/1 -> Relational Operator2/1
  Add2/1 -> Abs1/1
  RampLim1/1 -> Add2/2, MinMax1/2
  Constant6/1 -> RampLim1/4
  Constant5/1 -> RampLim1/3
  Switch3/1 -> Switch4/3, RampLim1/1
  Constant3/1 -> Switch3/1
  bool_OverrideSwitch/1 -> Switch3/2, Logical Operator1/1, Detect Decrease1/1
  Relational Operator2/1 -> S-R Flip-Flop1/2
  Detect Decrease1/1 -> S-R Flip-Flop1/1
  S-R Flip-Flop1/1 -> Logical Operator1/2
  S-R Flip-Flop1/2 -> Terminator1/1
  MinMax1/1 -> Switch4/1
  Unit Delay2/1 -> RampLim1/2
  Constant1/1 -> Switch2/2
  Switch2/1 -> bar_BrkPedlPModif/1

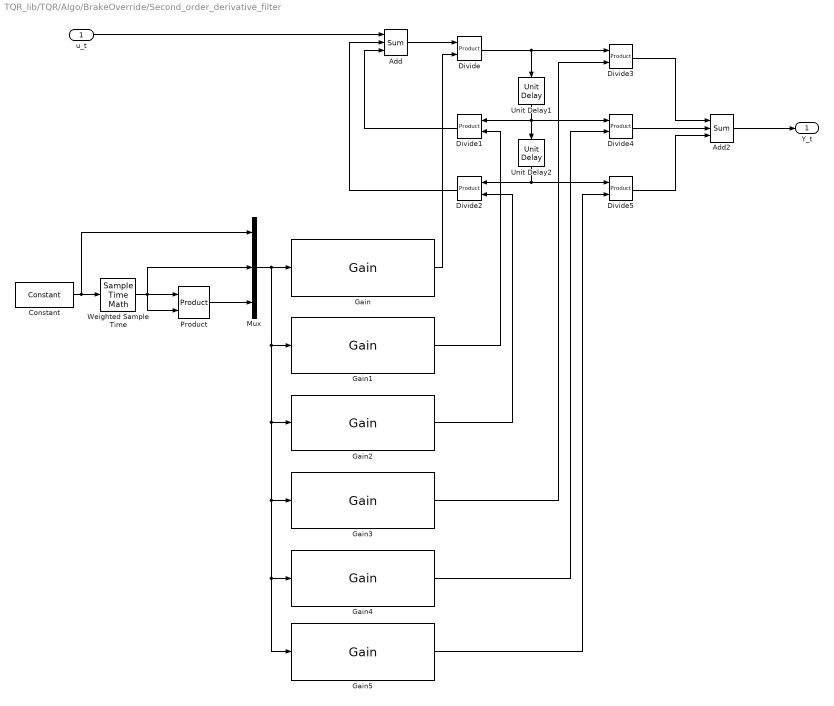
== system TQR_lib/TQR/Algo/BrakeOverride/Second_order_derivative_filter ==
  u_t : Inport
  Add : BaseOperationLib_Browser/Math Operations Changed/Sum  Inputs=+--  OutMin=[]  OutMax=[]  OutDataType=fixdt(1, 16)  OutScaling=2^0  OutDataTypeStr=Inherit: Inherit via back propagation
  Add2 : BaseOperationLib_Browser/Math Operations Changed/Sum  Inputs=+++  OutMin=[]  OutMax=[]  OutDataType=fixdt(1, 16)  OutScaling=2^0
  Constant : BaseOperationLib_Browser/Sources&Sinks/Constant  Value=1  OutMin=[]  OutMax=[]  OutDataTypeMode=single  OutDataType=fixdt(1, 16)  ConRadixGroup=Use specified scaling  OutScaling=2^0  OutDataTypeStr=single
  Divide : BaseOperationLib_Browser/Math Operations Changed/Product  Inputs=*/  Multiplication=Element-wise(.*)  OutMin=[]  OutMax=[]  OutDataType=fixdt(1,16,0)  OutScaling=[]
  Divide{1..5} (5 alike) : BaseOperationLib_Browser/Math Operations Changed/Product  Inputs=**  Multiplication=Element-wise(.*)  OutMin=[]  OutMax=[]  OutDataType=fixdt(1,16,0)  OutScaling=[]
  Gain : BaseOperationLib_Browser/Math Operations Changed/Gain  Gain=p1_ACPI_PICFilDen1_na  Multiplication=Matrix(K*u)  ParamMin=[]  ParamMax=[]  ParameterDataType=fixdt(1, 16)  ParameterScalingMode=Best Precision: Matrix-wise  ParameterScaling=2^0  ParamDataTypeStr=Inherit: Inherit from 'Gain'  OutMin=[]  OutMax=[]  OutDataType=fixdt(1, 16)  OutScaling=2^0  SaturateOnIntegerOverflow=on
  Gain1 : BaseOperationLib_Browser/Math Operations Changed/Gain  Gain=p1_ACPI_PICFilDen2_na  Multiplication=Matrix(K*u)  ParamMin=[]  ParamMax=[]  ParameterDataType=fixdt(1, 16)  ParameterScalingMode=Best Precision: Matrix-wise  ParameterScaling=2^0  ParamDataTypeStr=Inherit: Inherit from 'Gain'  OutMin=[]  OutMax=[]  OutDataType=fixdt(1, 16)  OutScaling=2^0  SaturateOnIntegerOverflow=on
  Gain2 : BaseOperationLib_Browser/Math Operations Changed/Gain  Gain=p1_ACPI_PICFilDen3_na  Multiplication=Matrix(K*u)  ParamMin=[]  ParamMax=[]  ParameterDataType=fixdt(1, 16)  ParameterScalingMode=Best Precision: Matrix-wise  ParameterScaling=2^0  ParamDataTypeStr=Inherit: Inherit from 'Gain'  OutMin=[]  OutMax=[]  OutDataType=fixdt(1, 16)  OutScaling=2^0  SaturateOnIntegerOverflow=on
  Gain3 : BaseOperationLib_Browser/Math Operations Changed/Gain  Gain=p1_ACPI_PICFilNum1_na  Multiplication=Matrix(K*u)  ParamMin=[]  ParamMax=[]  ParameterDataType=fixdt(1, 16)  ParameterScalingMode=Best Precision: Matrix-wise  ParameterScaling=2^0  ParamDataTypeStr=Inherit: Inherit from 'Gain'  OutMin=[]  OutMax=[]  OutDataType=fixdt(1, 16)  OutScaling=2^0  SaturateOnIntegerOverflow=on
  Gain4 : BaseOperationLib_Browser/Math Operations Changed/Gain  Gain=p1_ACPI_PICFilNum2_na  Multiplication=Matrix(K*u)  ParamMin=[]  ParamMax=[]  ParameterDataType=fixdt(1, 16)  ParameterScalingMode=Best Precision: Matrix-wise  ParameterScaling=2^0  ParamDataTypeStr=Inherit: Inherit from 'Gain'  OutMin=[]  OutMax=[]  OutDataType=fixdt(1, 16)  OutScaling=2^0  SaturateOnIntegerOverflow=on
  Gain5 : BaseOperationLib_Browser/Math Operations Changed/Gain  Gain=p1_ACPI_PICFilNum3_na  Multiplication=Matrix(K*u)  ParamMin=[]  ParamMax=[]  ParameterDataType=fixdt(1, 16)  ParameterScalingMode=Best Precision: Matrix-wise  ParameterScaling=2^0  ParamDataTypeStr=Inherit: Inherit from 'Gain'  OutMin=[]  OutMax=[]  OutDataType=fixdt(1, 16)  OutScaling=2^0  SaturateOnIntegerOverflow=on
  Mux : Mux  Inputs=3
  Product : BaseOperationLib_Browser/Math Operations Changed/Product  Inputs=2  Multiplication=Element-wise(.*)  OutMin=[]  OutMax=[]  OutDataTypeMode=single  OutDataType=fixdt(1,16,0)  OutScaling=[]  OutDataTypeStr=single  RndMeth=Zero  SaturateOnIntegerOverflow=on
  Unit Delay1 : BaseOperationLib_Browser/Discrete Unchanged /Unit Delay  X0=0  SampleTime=-1
  Unit Delay2 : BaseOperationLib_Browser/Discrete Unchanged /Unit Delay  X0=0  SampleTime=-1
  Weighted Sample Time : SampleTimeMath  TsampMathOp=Ts Only  OutDataTypeStr=Inherit: Inherit via back propagation
  Y_t : Outport
  wires:
  Add/1 -> Divide/1
  Unit Delay1/1 -> Unit Delay2/1, Divide1/1, Divide4/1
  Divide1/1 -> Add/3
  Divide2/1 -> Add/2
  Unit Delay2/1 -> Divide2/1, Divide5/1
  Divide4/1 -> Add2/2
  Divide/1 -> Unit Delay1/1, Divide3/1
  Divide5/1 -> Add2/3
  Divide3/1 -> Add2/1
  Add2/1 -> Y_t/1
  u_t/1 -> Add/1
  Weighted Sample Time/1 -> Mux/2, Product/1, Product/2
  Constant/1 -> Weighted Sample Time/1, Mux/1
  Product/1 -> Mux/3
  Mux/1 -> Gain/1, Gain1/1, Gain3/1, Gain5/1, Gain4/1, Gain2/1
  Gain/1 -> Divide/2
  Gain1/1 -> Divide1/2
  Gain2/1 -> Divide2/2
  Gain3/1 -> Divide3/2
  Gain4/1 -> Divide4/2
  Gain5/1 -> Divide5/2

== system TQR_lib/TQR/Algo/DrivabilityFilter/DrivingFilter ==
  Nm_TorqRateLimit : Inport
  pct_AccrPedlVal : Inport  Port=2
  bool_BrkPedlPsd : Inport  Port=3
  bar_BrkPedlP : Inport  Port=4
  kmph_VehLgtSpd : Inport  Port=5
  s_ShftLvrDly : Inport  Port=6
  bool_VehStandStillSts : Inport  Port=7
  Add3 : BaseOperationLib_Browser/Math Operations Changed/Sum  Inputs=-+  OutMin=[]  OutMax=[]  OutDataType=fixdt(1, 16)  OutScaling=2^0
  Compare To Constant3 : BaseOperationLib_Browser/Logic Operations Changed/Compare To Constant  SystemSampleTime=-1  relop=>=  const=p_single_Zero_M
  NormalFilter : Subsystem
  Switch10 : BaseOperationLib_Browser/Signal Routing Changed/Switch  Criteria=u2 ~= 0  Threshold=0  OutMin=[]  OutMax=[]  OutDataType=fixdt(1,16,0)  OutScaling=[]
  Unit Delay : BaseOperationLib_Browser/Discrete Unchanged /Unit Delay  X0=0  SampleTime=-1
  WerghtingFilter : BaseOperationLib_Browser/Discontinuities Unchanged/WerghtingFilter  SystemSampleTime=-1
  Nm_FilterTorqReq : Outport
  r_DrivingFilterFactor : Outport  Port=2
  wires:
  Nm_TorqRateLimit/1 -> WerghtingFilter/1, Add3/2
  WerghtingFilter/1 -> Nm_FilterTorqReq/1, Unit Delay/1
  Add3/1 -> Compare To Constant3/1
  Compare To Constant3/1 -> Switch10/2
  Switch10/1 -> WerghtingFilter/3, r_DrivingFilterFactor/1
  bar_BrkPedlP/1 -> NormalFilter/1(bar_BrkPedlP)
  bool_BrkPedlPsd/1 -> NormalFilter/3(bool_BrkPedlPsd)
  kmph_VehLgtSpd/1 -> NormalFilter/4(kmph_VehLgtSpd)
  s_ShftLvrDly/1 -> NormalFilter/5(s_ShftLvrDly)
  bool_VehStandStillSts/1 -> NormalFilter/6(bool_VehStandStillSts)
  pct_AccrPedlVal/1 -> NormalFilter/2(pct_AccrPedlVal)
  Unit Delay/1 -> WerghtingFilter/2, Add3/1
  NormalFilter/1(r_NormUppFilterFac) -> Switch10/1
  NormalFilter/2(r_NormDwnFilterFac) -> Switch10/3

== system TQR_lib/TQR/Algo/DrivabilityFilter/TorqRateLimit ==
  Nm_TorqueRaw : Inport
  bool_CrsCtlActive : Inport  Port=2
  pct_AccrPedlVal : Inport  Port=3
  Constant2 : BaseOperationLib_Browser/Sources&Sinks/Constant  Value=pTQR_Nmps_CrsCtlLowrRateLim_C  OutMin=[]  OutMax=[]  OutDataType=fixdt(1, 16)  ConRadixGroup=Use specified scaling  OutScaling=2^0  OutDataTypeStr=Inherit: Inherit from 'Constant value'
  Constant4 : BaseOperationLib_Browser/Sources&Sinks/Constant  Value=pTQR_Nmps_CrsCtlUpprRateLim_C  OutMin=[]  OutMax=[]  OutDataType=fixdt(1, 16)  ConRadixGroup=Use specified scaling  OutScaling=2^0  OutDataTypeStr=Inherit: Inherit from 'Constant value'
  LowrRateLimTable : BaseOperationLib_Browser/Lookup Tables Changed/Lookup Table  InputValues=pTQR_Nmps_AccPedValLowrRateLim_CUR  Table=pTQR_Nmps_LowrRateLimLoTbl_TAB  LookUpMeth=Interpolation-Use End Values  OutMin=[]  OutMax=[]  OutDataType=fixdt(1, 16)  OutScaling=2^0  OutDataTypeStr=Inherit: Inherit via back propagation  SaturateOnIntegerOverflow=on
      settings: AttributesFormatString=X:%<InputValues>\nTAB:%<Table>
  Rate Limiter Dynamic : BaseOperationLib_Browser/Discontinuities Unchanged/Rate Limiter Dynamic  SystemSampleTime=-1
  Switch3 : BaseOperationLib_Browser/Signal Routing Changed/Switch  Criteria=u2 ~= 0  Threshold=0  OutMin=[]  OutMax=[]  OutDataType=fixdt(1,16,0)  OutScaling=[]
  Switch7 : BaseOperationLib_Browser/Signal Routing Changed/Switch  Criteria=u2 ~= 0  Threshold=0  OutMin=[]  OutMax=[]  OutDataType=fixdt(1,16,0)  OutScaling=[]
  UpprRateLimTable : BaseOperationLib_Browser/Lookup Tables Changed/Lookup Table  InputValues=pTQR_Nmps_AccPedValUpprRateLim_CUR  Table=pTQR_Nmps_UpprRateLimLoTbl_TAB  LookUpMeth=Interpolation-Use End Values  OutMin=[]  OutMax=[]  OutDataType=fixdt(1, 16)  OutScaling=2^0  OutDataTypeStr=Inherit: Inherit via back propagation  SaturateOnIntegerOverflow=on
      settings: AttributesFormatString=X:%<InputValues>\nTAB:%<Table>
  Nm_TorqRateLimit : Outport
  wires:
  pct_AccrPedlVal/1 -> UpprRateLimTable/1, LowrRateLimTable/1
  Constant4/1 -> Switch3/1
  Constant2/1 -> Switch7/1
  Switch3/1 -> Rate Limiter Dynamic/1  "pTQR_Nmps_UpprRateLimMem"
  Switch7/1 -> Rate Limiter Dynamic/3  "pTQR_Nmps_LowrRateLimMem"
  LowrRateLimTable/1 -> Switch7/3
  UpprRateLimTable/1 -> Switch3/3
  bool_CrsCtlActive/1 -> Switch3/2, Switch7/2
  Nm_TorqueRaw/1 -> Rate Limiter Dynamic/2
  Rate Limiter Dynamic/1 -> Nm_TorqRateLimit/1
